simulink model "controle_estabilidade_magnetorquer_e_rw_4"  (R2021b)
settings: Solver=ode45  StartTime=0.0  StopTime=5000  MaxStep=0.4  RelTol=1e-3
values from neighbouring files (symbols this model uses):
  A = 1    [parametros2.mat]
  b = 5.16e-06    [parametros.mat]    (also in parametros2.mat)
  J = [0.00216966666667  0  0; 0  0.00216966666667  0; 0  0  0.00216966666667]    [parametros.mat]    (also in parametros2.mat)
  n = 100    [parametros2.mat]
undefined symbols (not defined in the file or in its folder): Jm, K, L, R
libraries: matrix_library x3, aerolibutil x2, slpidlib x2, sharedutil x2
settings Model: Creator=JRRL  LastModifiedBy=JRRL

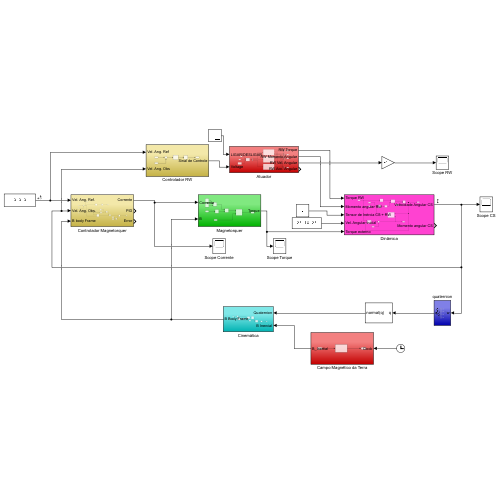
[thumbnail: Simulink's stored preview of the top-level diagram]
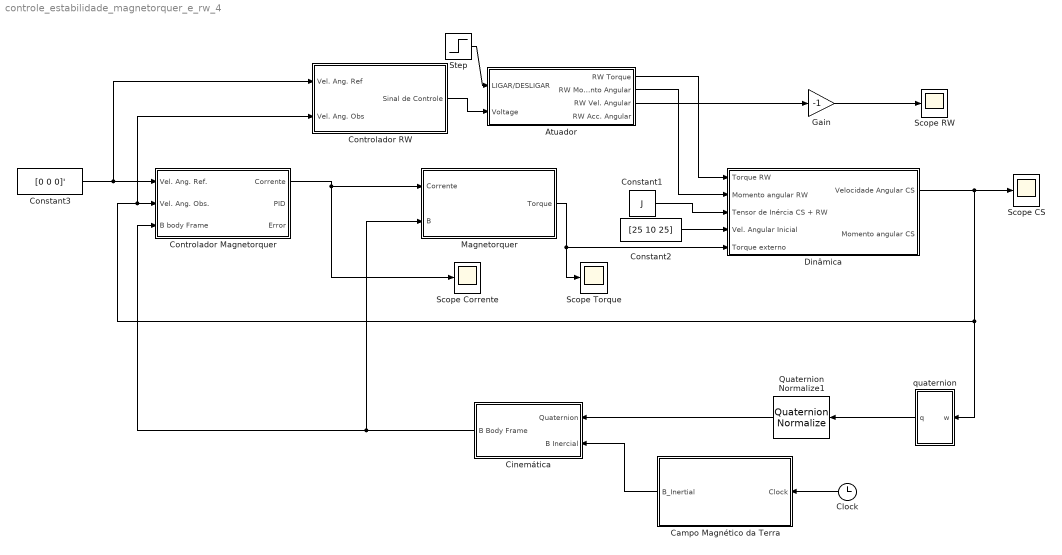
== system controle_estabilidade_magnetorquer_e_rw_4 ==
  Atuador : Subsystem
  Campo Magnético da Terra : Subsystem
  Cinemática : Subsystem
  Clock : Clock
  Constant1 : Constant  Value=J
  Constant2 : Constant  Value=[25 10 25]
  Constant3 : Constant  Value=[0 0 0]'
  Controlador Magnetorquer : Subsystem
  Controlador RW : Subsystem
  Dinâmica : Subsystem
  Gain : Gain  Gain=-1
  Magnetorquer : Subsystem
  Quaternion Normalize1 : sharedutil/Quaternion Normalize  aMode=aMode
      settings: SourceProductBaseCode=AE,PW,DR,MT,UV,VE
  Scope CS : Scope
  Scope Corrente : Scope
  Scope RW : Scope
  Scope Torque : Scope
  Step : Step  Time=3000  Before=1  After=0  SampleTime=0
  quaternion : Subsystem
  wires:
  Constant1/1 -> Dinâmica/3(Tensor de Inércia CS + RW)
  Constant2/1 -> Dinâmica/4(Vel. Angular Inicial)
  quaternion/1(q) -> Quaternion Normalize1/1
  Controlador Magnetorquer/1(Corrente) -> Scope Corrente/1, Magnetorquer/1(Corrente)
  Quaternion Normalize1/1 -> Cinemática/1(Quaternion)
  Magnetorquer/1(Torque) -> Dinâmica/5(Torque externo), Scope Torque/1
  Campo Magnético da Terra/1(B_Inertial) -> Cinemática/2(B Inercial)
  Cinemática/1(B Body Frame) -> Magnetorquer/2(B), Controlador Magnetorquer/3(B body Frame)
  Clock/1 -> Campo Magnético da Terra/1(Clock)
  Dinâmica/1(Velocidade Angular CS) -> Scope CS/1, quaternion/1(w), Controlador RW/2(Vel. Ang. Obs), Controlador Magnetorquer/2(Vel. Ang. Obs.)
  Constant3/1 -> Controlador RW/1(Vel. Ang. Ref), Controlador Magnetorquer/1(Vel. Ang. Ref.)
  Atuador/1(RW Torque) -> Dinâmica/1(Torque RW)
  Atuador/2(RW Momento Angular) -> Dinâmica/2(Momento angular RW)
  Controlador RW/1(Sinal de Controle) -> Atuador/2(Voltage)
  Step/1 -> Atuador/1(LIGAR/DESLIGAR)
  Atuador/3(RW Vel. Angular) -> Gain/1
  Gain/1 -> Scope RW/1

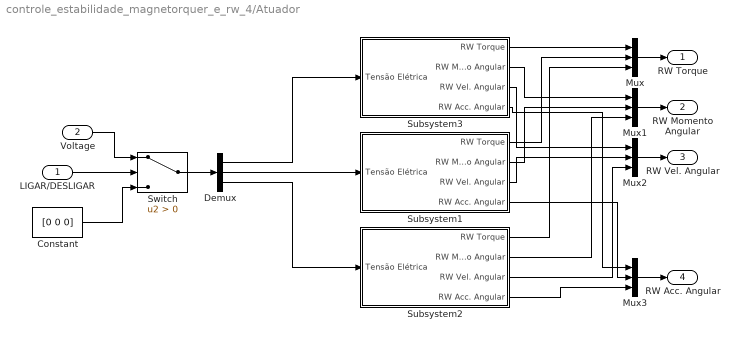
== system controle_estabilidade_magnetorquer_e_rw_4/Atuador ==
  LIGAR/DESLIGAR : Inport
  Voltage : Inport  Port=2
  Constant : Constant  Value=[0 0 0]
  Demux : Demux  Outputs=3
  Mux{,1..3} (4 alike) : Mux  Inputs=3
  Subsystem1 : Subsystem
  Subsystem2 : Subsystem
  Subsystem3 : Subsystem
  Switch : Switch  Criteria=u2 > Threshold
  RW Torque : Outport
  RW Momento Angular : Outport  Port=2
  RW Vel. Angular : Outport  Port=3
  RW Acc. Angular : Outport  Port=4
  wires:
  Switch/1 -> Demux/1
  Demux/1 -> Subsystem3/1(Tensão Elétrica)
  Demux/2 -> Subsystem1/1(Tensão Elétrica)
  Demux/3 -> Subsystem2/1(Tensão Elétrica)
  Subsystem3/1(RW Torque) -> Mux/1
  Subsystem1/1(RW Torque) -> Mux/2
  Subsystem2/1(RW Torque) -> Mux/3
  Subsystem3/2(RW Momento Angular) -> Mux1/1
  Subsystem1/2(RW Momento Angular) -> Mux1/2
  Subsystem2/2(RW Momento Angular) -> Mux1/3
  Subsystem3/3(RW Vel. Angular) -> Mux2/1
  Subsystem1/3(RW Vel. Angular) -> Mux2/2
  Subsystem2/3(RW Vel. Angular) -> Mux2/3
  Subsystem3/4(RW Acc. Angular) -> Mux3/1
  Subsystem1/4(RW Acc. Angular) -> Mux3/2
  Subsystem2/4(RW Acc. Angular) -> Mux3/3
  Mux/1 -> RW Torque/1
  Mux1/1 -> RW Momento Angular/1
  Mux2/1 -> RW Vel. Angular/1
  Mux3/1 -> RW Acc. Angular/1
  LIGAR/DESLIGAR/1 -> Switch/2
  Voltage/1 -> Switch/1
  Constant/1 -> Switch/3

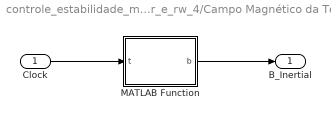
== system controle_estabilidade_magnetorquer_e_rw_4/Campo Magnético da Terra ==
  Clock : Inport
  MATLAB Function : MATLAB Function  TreatAsAtomicUnit=on
  B_Inertial : Outport
  wires:
  Clock/1 -> MATLAB Function/1(t)
  MATLAB Function/1(b) -> B_Inertial/1

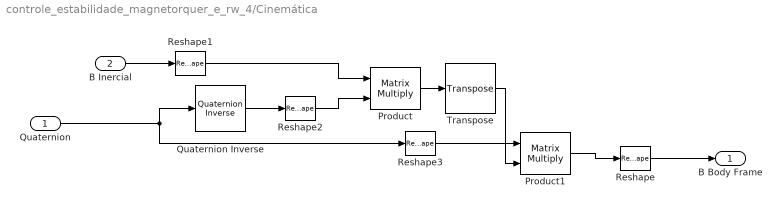
== system controle_estabilidade_magnetorquer_e_rw_4/Cinemática ==
  Quaternion : Inport
  B Inercial : Inport  Port=2
  Product : Product  Multiplication=Matrix(*)
  Product1 : Product  Multiplication=Matrix(*)
  Quaternion Inverse : aerolibutil/Quaternion Inverse
  Reshape : Reshape  OutputDimensionality=Column vector (2-D)
  Reshape1 : Reshape  OutputDimensionality=Column vector (2-D)
  Reshape2 : Reshape  OutputDimensionality=Row vector (2-D)
  Reshape3 : Reshape  OutputDimensionality=Row vector (2-D)
  Transpose : matrix_library/Transpose
      settings: SourceProductBaseCode=SL
  B Body Frame : Outport
  wires:
  Quaternion Inverse/1 -> Reshape2/1
  B Inercial/1 -> Reshape1/1
  Product1/1 -> Reshape/1
  Reshape/1 -> B Body Frame/1
  Reshape1/1 -> Product/1
  Reshape2/1 -> Product/2
  Quaternion/1 -> Reshape3/1, Quaternion Inverse/1
  Reshape3/1 -> Product1/1
  Product/1 -> Transpose/1
  Transpose/1 -> Product1/2

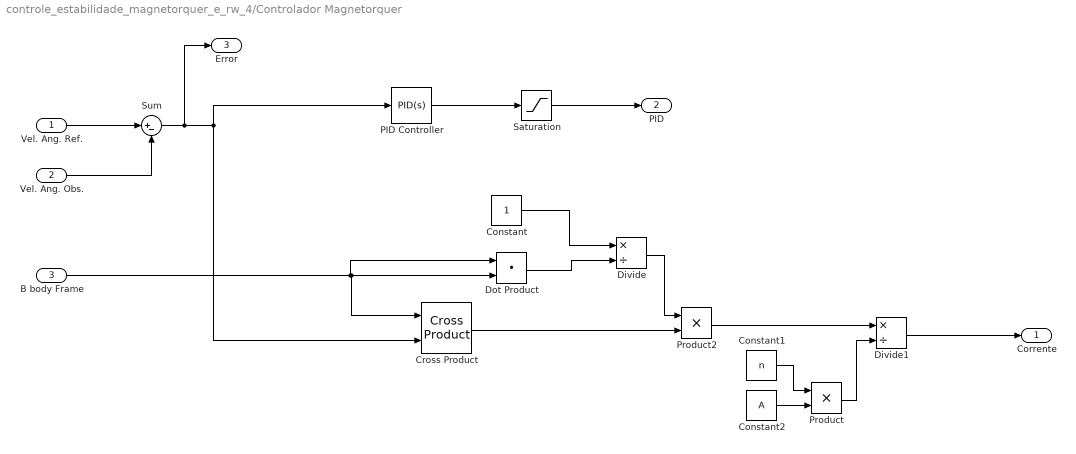
== system controle_estabilidade_magnetorquer_e_rw_4/Controlador Magnetorquer ==
  Vel. Ang. Ref. : Inport
  Vel. Ang. Obs. : Inport  Port=2
  B body Frame : Inport  Port=3
  Constant : Constant
  Constant1 : Constant  Value=n
  Constant2 : Constant  Value=A
  Cross Product : matrix_library/Cross Product
      settings: SourceProductBaseCode=SL
  Divide : Product  Inputs=*/
  Divide1 : Product  Inputs=*/
  Dot Product : DotProduct  InputSameDT=on  OutDataTypeStr=Inherit: Inherit via internal rule
  PID Controller : slpidlib/PID Controller  Controller=PID  Form=Parallel  TimeDomain=Continuous-time  UseExternalTs=off  SampleTime=-1  IntegratorMethod=Forward Euler  FilterMethod=Forward Euler  ControllerParametersSource=internal  P=1  I=0  D=0.1  UseFilter=on  N=100  TunerSelectOption=Transfer Function Based (PID Tuner App)  InitialConditionSource=internal  InitialConditionForIntegrator=0  InitialConditionForFilter=0  DifferentiatorICPrevScaledInput=0  ExternalReset=none  TrackingMode=off  Kt=1  LimitOutput=off  SatLimitsSource=internal  UpperSaturationLimit=inf  LowerSaturationLimit=-inf  LinearizeAsGain=on  AntiWindupMode=none  Kb=1  POutMin=[]  POutMax=[]  IOutMin=[]  IOutMax=[]  DOutMin=[]  DOutMax=[]  NOutMin=[]  NOutMax=[]  SumOutMin=[]  SumOutMax=[]  SaturationOutMin=[]  SaturationOutMax=[]  PParamMin=[]  PParamMax=[]  IParamMin=[]  IParamMax=[]  DParamMin=[]  DParamMax=[]  NParamMin=[]  NParamMax=[]  KbParamMin=[]  KbParamMax=[]  KtParamMin=[]  KtParamMax=[]  KbOutMin=[]  KbOutMax=[]  KtOutMin=[]  KtOutMax=[]  IntegratorOutMin=[]  IntegratorOutMax=[]  FilterOutMin=[]  FilterOutMax=[]  SumI1OutMin=[]  SumI1OutMax=[]  SumI2OutMin=[]  SumI2OutMax=[]  SumI3OutMin=[]  SumI3OutMax=[]  SumI4OutMin=[]  SumI4OutMax=[]  SumDOutMin=[]  SumDOutMax=[]  DifferentiatorOutMin=[]  DifferentiatorOutMax=[]  FilterDiffOutCoefMin=[]  FilterDiffOutCoefMax=[]  ReciprocalOutMin=[]  ReciprocalOutMax=[]  SumDenOutMin=[]  SumDenOutMax=[]  SumNumOutMin=[]  SumNumOutMax=[]  DivideOutMin=[]  DivideOutMax=[]  UdiffTsProdOutMin=[]  UdiffTsProdOutMax=[]  NTsProdOutMin=[]  NTsProdOutMax=[]  UintegralTsProdOutMin=[]  UintegralTsProdOutMax=[]  UngainTsProdOutMin=[]  UngainTsProdOutMax=[]  IntegratorContinuousStateAttributes=''  IntegratorStateMustResolveToSignalObject=off  IntegratorRTWStateStorageClass=Auto  FilterContinuousStateAttributes=''  FilterStateMustResolveToSignalObject=off  FilterRTWStateStorageClass=Auto  ParallelPVariant=InternalParameters  IdealPVariant=Disabled  IVariant=InternalParameters  DVariant=InternalParameters  IntegratorVariant=Continuous  SatVariant=Disabled  AWVariant=Passthrough  PCopyVariant=Disabled  TRVariant=Disabled  FdbkBlocksVariant=Forward  IdealPFdbkVariant=Disabled  SatFdbkVariant=Disabled  DerivativeFilterVariant=ContFilter  NVariant=InternalParameters  NCopyVariant=Disabled  FilterICVariant=InternalICsFilter  IntegratorICVariant=InternalICs  ExternalResetVariant=Disabled  TRSumVariant=Passthrough  SumFdbkVariant=Disabled  SumVariant=Sum_PID  TsampFilterVariant=InternalTs  TsampNgainVariant=Passthrough  TsampIntegralVariant=Passthrough  ExternalSaturationOutDataTypeStr=Inherit: Same as second input
  Product : Product
  Product2 : Product
  Saturation : Saturate  UpperLimit=1  LowerLimit=-1
  Sum : Sum  Inputs=|+-
  Corrente : Outport
  PID : Outport  Port=2
  Error : Outport  Port=3
  wires:
  Vel. Ang. Ref./1 -> Sum/1
  Vel. Ang. Obs./1 -> Sum/2
  Dot Product/1 -> Divide/2
  Cross Product/1 -> Product2/2
  Divide/1 -> Product2/1
  Sum/1 -> Error/1, PID Controller/1, Cross Product/2
  B body Frame/1 -> Dot Product/1, Dot Product/2, Cross Product/1
  Saturation/1 -> PID/1
  PID Controller/1 -> Saturation/1
  Constant1/1 -> Product/1
  Constant2/1 -> Product/2
  Product/1 -> Divide1/2
  Product2/1 -> Divide1/1
  Divide1/1 -> Corrente/1
  Constant/1 -> Divide/1

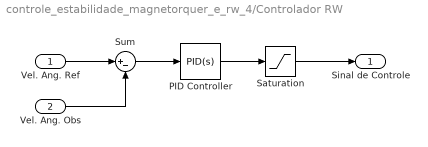
== system controle_estabilidade_magnetorquer_e_rw_4/Controlador RW ==
  Vel. Ang. Ref : Inport
  Vel. Ang. Obs : Inport  Port=2
  PID Controller : slpidlib/PID Controller  Controller=PID  Form=Parallel  TimeDomain=Continuous-time  UseExternalTs=off  SampleTime=-1  IntegratorMethod=Forward Euler  FilterMethod=Forward Euler  ControllerParametersSource=internal  P=1  I=1  D=0.1  UseFilter=on  N=100  TunerSelectOption=Transfer Function Based (PID Tuner App)  InitialConditionSource=internal  InitialConditionForIntegrator=0  InitialConditionForFilter=0  DifferentiatorICPrevScaledInput=0  ExternalReset=none  TrackingMode=off  Kt=1  LimitOutput=off  SatLimitsSource=internal  UpperSaturationLimit=inf  LowerSaturationLimit=-inf  LinearizeAsGain=on  AntiWindupMode=none  Kb=1  POutMin=[]  POutMax=[]  IOutMin=[]  IOutMax=[]  DOutMin=[]  DOutMax=[]  NOutMin=[]  NOutMax=[]  SumOutMin=[]  SumOutMax=[]  SaturationOutMin=[]  SaturationOutMax=[]  PParamMin=[]  PParamMax=[]  IParamMin=[]  IParamMax=[]  DParamMin=[]  DParamMax=[]  NParamMin=[]  NParamMax=[]  KbParamMin=[]  KbParamMax=[]  KtParamMin=[]  KtParamMax=[]  KbOutMin=[]  KbOutMax=[]  KtOutMin=[]  KtOutMax=[]  IntegratorOutMin=[]  IntegratorOutMax=[]  FilterOutMin=[]  FilterOutMax=[]  SumI1OutMin=[]  SumI1OutMax=[]  SumI2OutMin=[]  SumI2OutMax=[]  SumI3OutMin=[]  SumI3OutMax=[]  SumI4OutMin=[]  SumI4OutMax=[]  SumDOutMin=[]  SumDOutMax=[]  DifferentiatorOutMin=[]  DifferentiatorOutMax=[]  FilterDiffOutCoefMin=[]  FilterDiffOutCoefMax=[]  ReciprocalOutMin=[]  ReciprocalOutMax=[]  SumDenOutMin=[]  SumDenOutMax=[]  SumNumOutMin=[]  SumNumOutMax=[]  DivideOutMin=[]  DivideOutMax=[]  UdiffTsProdOutMin=[]  UdiffTsProdOutMax=[]  NTsProdOutMin=[]  NTsProdOutMax=[]  UintegralTsProdOutMin=[]  UintegralTsProdOutMax=[]  UngainTsProdOutMin=[]  UngainTsProdOutMax=[]  IntegratorContinuousStateAttributes=''  IntegratorStateMustResolveToSignalObject=off  IntegratorRTWStateStorageClass=Auto  FilterContinuousStateAttributes=''  FilterStateMustResolveToSignalObject=off  FilterRTWStateStorageClass=Auto  ParallelPVariant=InternalParameters  IdealPVariant=Disabled  IVariant=InternalParameters  DVariant=InternalParameters  IntegratorVariant=Continuous  SatVariant=Disabled  AWVariant=Passthrough  PCopyVariant=Disabled  TRVariant=Disabled  FdbkBlocksVariant=Forward  IdealPFdbkVariant=Disabled  SatFdbkVariant=Disabled  DerivativeFilterVariant=ContFilter  NVariant=InternalParameters  NCopyVariant=Disabled  FilterICVariant=InternalICsFilter  IntegratorICVariant=InternalICs  ExternalResetVariant=Disabled  TRSumVariant=Passthrough  SumFdbkVariant=Disabled  SumVariant=Sum_PID  TsampFilterVariant=InternalTs  TsampNgainVariant=Passthrough  TsampIntegralVariant=Passthrough  ExternalSaturationOutDataTypeStr=Inherit: Same as second input
  Saturation : Saturate  UpperLimit=12  LowerLimit=-12
  Sum : Sum  Inputs=|+-
  Sinal de Controle : Outport
  wires:
  Vel. Ang. Ref/1 -> Sum/1
  Vel. Ang. Obs/1 -> Sum/2
  Sum/1 -> PID Controller/1
  PID Controller/1 -> Saturation/1
  Saturation/1 -> Sinal de Controle/1

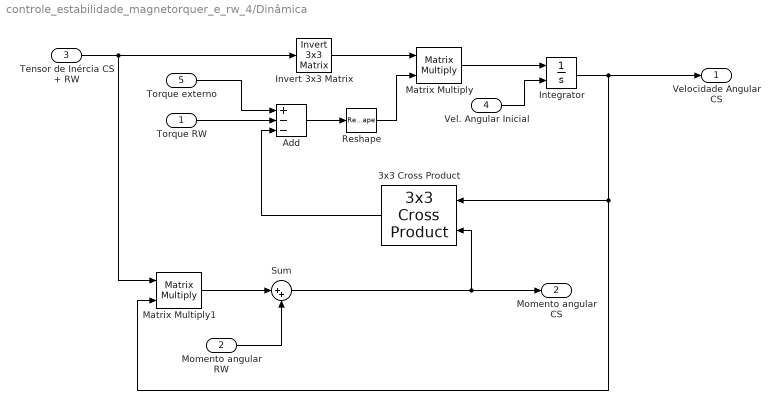
== system controle_estabilidade_magnetorquer_e_rw_4/Dinâmica ==
  Torque RW : Inport
  Momento angular RW : Inport  Port=2
  Tensor de Inércia CS + RW : Inport  Port=3
  Vel. Angular Inicial : Inport  Port=4
  Torque externo : Inport  Port=5
  3x3 Cross Product : sharedutil/3x3 Cross Product  aMode=aMode
      settings: SourceProductBaseCode=AE,PW,DR,MT,UV,VE
  Add : Sum  Inputs=+--
  Integrator : Integrator  InitialConditionSource=external
  Invert 3x3 Matrix : aerolibutil/Invert  3x3 Matrix
  Matrix Multiply : Product  Multiplication=Matrix(*)
  Matrix Multiply1 : Product  Multiplication=Matrix(*)
  Reshape : Reshape  OutputDimensionality=Column vector (2-D)
  Sum : Sum  Inputs=|++
  Velocidade Angular CS : Outport
  Momento angular CS : Outport  Port=2
  wires:
  Sum/1 -> Momento angular CS/1, 3x3 Cross Product/2
  3x3 Cross Product/1 -> Add/3
  Invert 3x3 Matrix/1 -> Matrix Multiply/1
  Integrator/1 -> Velocidade Angular CS/1, Matrix Multiply1/2, 3x3 Cross Product/1
  Matrix Multiply/1 -> Integrator/1
  Momento angular RW/1 -> Sum/2
  Torque RW/1 -> Add/2
  Tensor de Inércia CS + RW/1 -> Matrix Multiply1/1, Invert 3x3 Matrix/1
  Torque externo/1 -> Add/1
  Vel. Angular Inicial/1 -> Integrator/2
  Add/1 -> Reshape/1
  Matrix Multiply1/1 -> Sum/1
  Reshape/1 -> Matrix Multiply/2

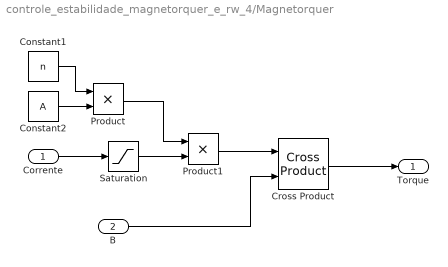
== system controle_estabilidade_magnetorquer_e_rw_4/Magnetorquer ==
  Corrente : Inport
  B : Inport  Port=2
  Constant1 : Constant  Value=n
  Constant2 : Constant  Value=A
  Cross Product : matrix_library/Cross Product
      settings: SourceProductBaseCode=SL
  Product : Product
  Product1 : Product
  Saturation : Saturate
  Torque : Outport
  wires:
  B/1 -> Cross Product/2
  Cross Product/1 -> Torque/1
  Corrente/1 -> Saturation/1
  Constant2/1 -> Product/2
  Constant1/1 -> Product/1
  Saturation/1 -> Product1/2
  Product/1 -> Product1/1
  Product1/1 -> Cross Product/1

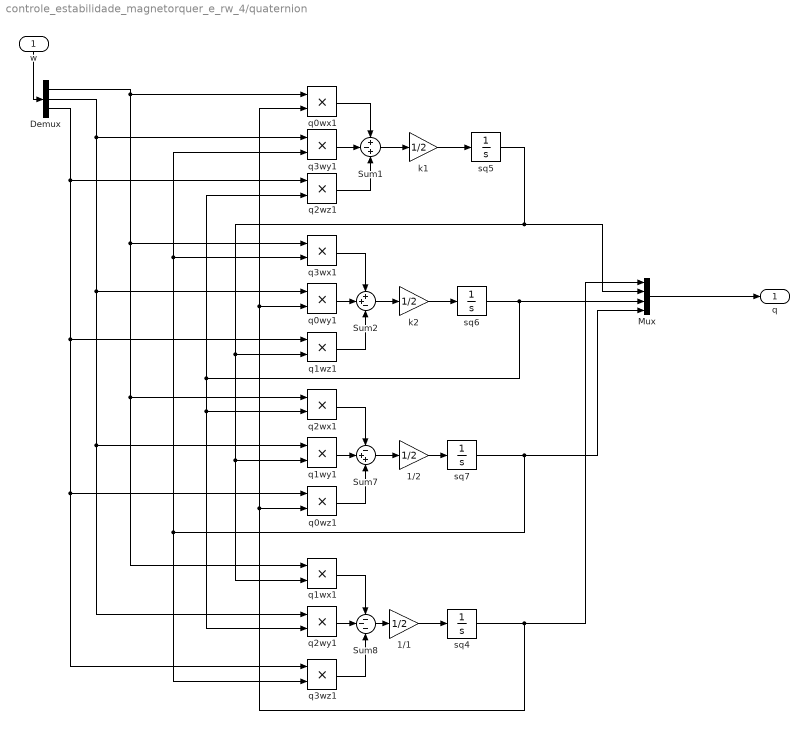
== system controle_estabilidade_magnetorquer_e_rw_4/quaternion ==
  w : Inport
  1/1 : Gain  Gain=1/2
  1/2 : Gain  Gain=1/2
  Demux : Demux  Outputs=3
  Mux : Mux
  Sum1 : Sum  Inputs=+-+
  Sum2 : Sum  Inputs=++-
  Sum7 : Sum  Inputs=-++
  Sum8 : Sum  Inputs=---
  k1 : Gain  Gain=1/2
  k2 : Gain  Gain=1/2
  q0wx1 : Product  RndMeth=Zero
  q0wy1 : Product  RndMeth=Zero
  q0wz1 : Product  RndMeth=Zero
  q1wx1 : Product  RndMeth=Zero
  q1wy1 : Product  RndMeth=Zero
  q1wz1 : Product  RndMeth=Zero
  q2wx1 : Product  RndMeth=Zero
  q2wy1 : Product  RndMeth=Zero
  q2wz1 : Product  RndMeth=Zero
  q3wx1 : Product  RndMeth=Zero
  q3wy1 : Product  RndMeth=Zero
  q3wz1 : Product  RndMeth=Zero
  sq4 : Integrator  InitialCondition=1
  sq5 : Integrator
  sq6 : Integrator
  sq7 : Integrator
  q : Outport
  wires:
  Sum1/1 -> k1/1
  sq5/1 -> q1wx1/2, q1wy1/2, q1wz1/2, Mux/2
  1/2/1 -> sq7/1
  q3wz1/1 -> Sum8/3
  q0wz1/1 -> Sum7/3
  sq6/1 -> q2wy1/2, q2wx1/2, q2wz1/2, Mux/3
  sq7/1 -> q3wz1/2, q3wx1/2, q3wy1/2, Mux/4
  Demux/1 -> q1wx1/1, q2wx1/1, q3wx1/1, q0wx1/1
  k1/1 -> sq5/1
  q3wy1/1 -> Sum1/2
  q2wx1/1 -> Sum7/1
  q0wx1/1 -> Sum1/1
  k2/1 -> sq6/1
  Sum7/1 -> 1/2/1
  Demux/3 -> q3wz1/1, q0wz1/1, q1wz1/1, q2wz1/1
  Demux/2 -> q2wy1/1, q1wy1/1, q0wy1/1, q3wy1/1
  Sum2/1 -> k2/1
  sq4/1 -> q0wz1/2, q0wy1/2, q0wx1/2, Mux/1
  q1wz1/1 -> Sum2/3
  1/1/1 -> sq4/1
  q2wy1/1 -> Sum8/2
  q2wz1/1 -> Sum1/3
  q0wy1/1 -> Sum2/2
  q1wx1/1 -> Sum8/1
  w/1 -> Demux/1
  Mux/1 -> q/1
  Sum8/1 -> 1/1/1
  q1wy1/1 -> Sum7/2
  q3wx1/1 -> Sum2/1

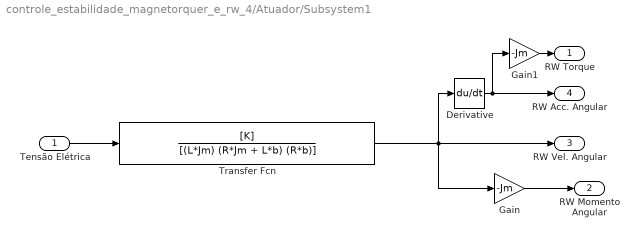
== system controle_estabilidade_magnetorquer_e_rw_4/Atuador/Subsystem1 ==
  Tensão Elétrica : Inport
  Derivative : Derivative
  Gain : Gain  Gain=-Jm
  Gain1 : Gain  Gain=-Jm
  Transfer Fcn : TransferFcn  Numerator=[K]  Denominator=[(L*Jm) (R*Jm + L*b) (R*b)]
  RW Torque : Outport
  RW Momento Angular : Outport  Port=2
  RW Vel. Angular : Outport  Port=3
  RW Acc. Angular : Outport  Port=4
  wires:
  Tensão Elétrica/1 -> Transfer Fcn/1
  Transfer Fcn/1 -> Gain/1, Derivative/1, RW Vel. Angular/1
  Gain/1 -> RW Momento Angular/1
  Derivative/1 -> RW Acc. Angular/1, Gain1/1
  Gain1/1 -> RW Torque/1

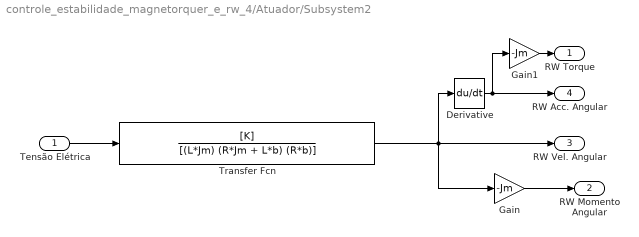
== system controle_estabilidade_magnetorquer_e_rw_4/Atuador/Subsystem2 ==
  Tensão Elétrica : Inport
  Derivative : Derivative
  Gain : Gain  Gain=-Jm
  Gain1 : Gain  Gain=-Jm
  Transfer Fcn : TransferFcn  Numerator=[K]  Denominator=[(L*Jm) (R*Jm + L*b) (R*b)]
  RW Torque : Outport
  RW Momento Angular : Outport  Port=2
  RW Vel. Angular : Outport  Port=3
  RW Acc. Angular : Outport  Port=4
  wires:
  Tensão Elétrica/1 -> Transfer Fcn/1
  Transfer Fcn/1 -> Gain/1, Derivative/1, RW Vel. Angular/1
  Gain/1 -> RW Momento Angular/1
  Derivative/1 -> RW Acc. Angular/1, Gain1/1
  Gain1/1 -> RW Torque/1

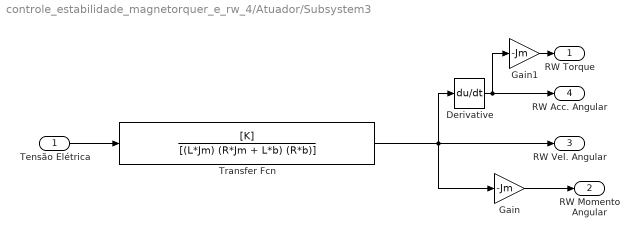
== system controle_estabilidade_magnetorquer_e_rw_4/Atuador/Subsystem3 ==
  Tensão Elétrica : Inport
  Derivative : Derivative
  Gain : Gain  Gain=-Jm
  Gain1 : Gain  Gain=-Jm
  Transfer Fcn : TransferFcn  Numerator=[K]  Denominator=[(L*Jm) (R*Jm + L*b) (R*b)]
  RW Torque : Outport
  RW Momento Angular : Outport  Port=2
  RW Vel. Angular : Outport  Port=3
  RW Acc. Angular : Outport  Port=4
  wires:
  Tensão Elétrica/1 -> Transfer Fcn/1
  Transfer Fcn/1 -> Gain/1, Derivative/1, RW Vel. Angular/1
  Gain/1 -> RW Momento Angular/1
  Derivative/1 -> RW Acc. Angular/1, Gain1/1
  Gain1/1 -> RW Torque/1

== matlab function controle_estabilidade_magnetorquer_e_rw_4/Campo Magnético da Terra/MATLAB Function ==
  data: t input; b output
function b = fcn(t)    
    b = (1/(2*(t+1)))*[t+2, sqrt(3*t*t + 4*t)*sin(t),sqrt(3*t*t+4*t)*cos(t)];
